simulink model "SimulinkRobot_Test1_GravityCompensation"  (R2023b)
settings: Solver=VariableStepAuto  StartTime=0.0  StopTime=5  RelTol=1e-3
values from neighbouring files (symbols this model uses):
  grav = [0 0 0 0 0 -9.8]    [UR5_Data.mat]
  Mlist = [0.0102675 0 0 0 0 0 0 0.0102675 0 0 0 0 ... (216 elements, 6x6x6)]    [UR5_Data.mat]
  TfLists = [1 0 0 0 0 1 0 0 0 0 1 0 ... (112 elements, 4x4x7)]    [UR5_Data.mat]    (also in UR5_Regressor.mat)
  Twists = [xi1',xi2',xi3',xi4',xi5',xi6']    [Example1_InvKin.m]    (also in UR5_Data.mat = [0 0 1 0 0 0 0 1 0 -0.089 0 0 ... (36 elements, 6x6)]; UR5_Regressor.mat = [0 0 1 0 0 0 0 1 0 -0.089 0 0 ... (36 elements, 6x6)])
settings Model: Creator=mechmedic  LastModifiedBy=mechmedic

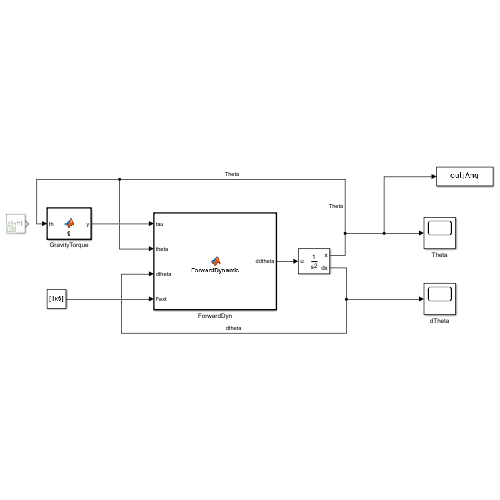
[thumbnail: Simulink's stored preview of the top-level diagram]
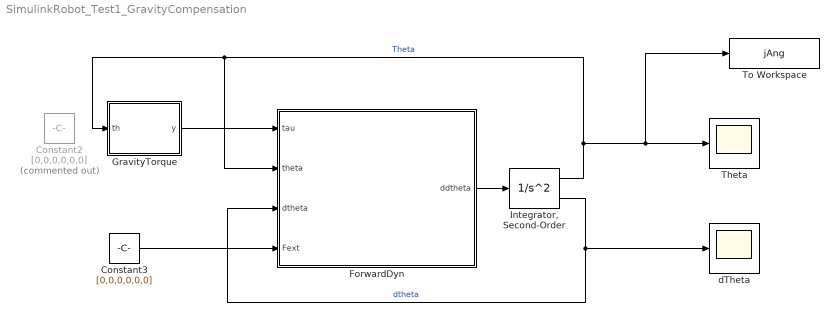
== system SimulinkRobot_Test1_GravityCompensation ==
  Constant2 : Constant  Commented=on  Value=[0,0,0,0,0,0]
  Constant3 : Constant  Value=[0,0,0,0,0,0]
  ForwardDyn : MATLAB Function  TreatAsAtomicUnit=on
  GravityTorque : MATLAB Function  TreatAsAtomicUnit=on
  "Integrator, Second-Order" : SecondOrderIntegrator
  Theta : Scope
  To Workspace : ToWorkspace  VariableName=jAng  SaveFormat=Timeseries  SampleTime=-1
  dTheta : Scope
  wires:
  Constant3/1 -> ForwardDyn/4(Fext)
  ForwardDyn/1(ddtheta) -> "Integrator, Second-Order"/1
  "Integrator, Second-Order"/1 -> GravityTorque/1(th), ForwardDyn/2(theta), To Workspace/1, Theta/1  "Theta"
  "Integrator, Second-Order"/2 -> dTheta/1, ForwardDyn/3(dtheta)  "dtheta"
  GravityTorque/1(y) -> ForwardDyn/1(tau)

== matlab function SimulinkRobot_Test1_GravityCompensation/GravityTorque ==
  data: th input; y output; Twists parameter; TfLists parameter; Mlist parameter; grav parameter
function y = g(th,Twists, TfLists, Mlist, grav)
    y = GravityTorque(th, Twists, TfLists, Mlist, grav);

== matlab function SimulinkRobot_Test1_GravityCompensation/ForwardDyn ==
  settings: sampleTime=0.01
  data: tau input size=[6 1]; theta input double size=[6 1]; dtheta input double size=[6 1]; Fext input; Twists parameter size=size(Twists); TfLists parameter size=size(TfLists); ddtheta output double size=[6 1]; Mlist parameter size=size(Mlist); grav parameter size=size(grav)
function ddtheta =  ForwardDynamic (tau, theta, dtheta, Fext, Twists, TfLists, Mlist, grav)
    ddtheta =  FwdDyn(tau, theta, dtheta, Fext, Twists, TfLists, Mlist, grav);
